simulink library "INT_WESDem_SetPoint"  (R2016b)
settings: Solver=VariableStepAuto  StartTime=0.0  StopTime=10.0  RelTol=1e-3
settings Model: Creator=zhoukai  LastModifiedBy=zhoukai

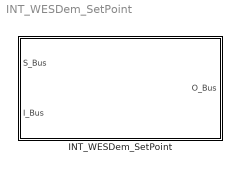
== system INT_WESDem_SetPoint ==
  INT_WESDem_SetPoint : Subsystem

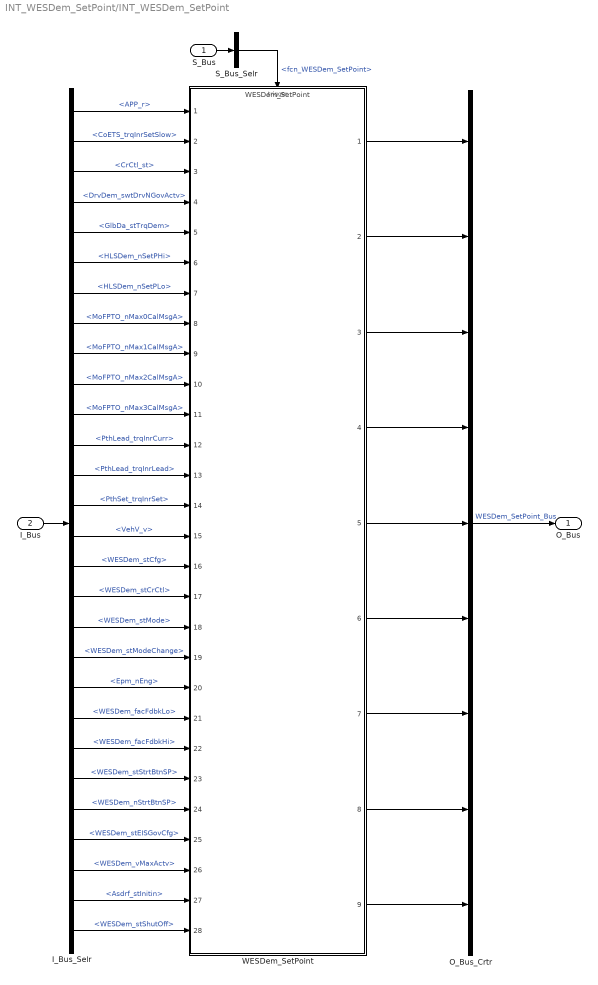
== system INT_WESDem_SetPoint/INT_WESDem_SetPoint ==
  S_Bus : Inport
  I_Bus : Inport  Port=2
  I_Bus_Selr : BusSelector  OutputSignals=APP_r,CoETS_trqInrSetSlow,CrCtl_st,DrvDem_swtDrvNGovActv,GlbDa_stTrqDem,HLSDem_nSetPHi,HLSDem_nSetPLo,MoFPTO_nMax0CalMsgA,MoFPTO_nMax1CalMsgA,MoFPTO_nMax2CalMsgA,MoFPTO_nMax3CalMsgA,PthLead_trqInrCurr,PthLead_trqInrLead,PthSet_trqInrSet,VehV_v,WESDem_stCfg,WESDem_stCrCtl,WESDem_stMode,WESDem_stModeChange,Epm_nEng,WESDem_facFdbkLo,WESDem_facFdbkHi,WESDem_stStrtBtnSP,WESDem_nStrtBtnSP,WESDem_stEISGovCfg,WESDem_vMaxActv,Asdrf_stInitin,WESDem_stShutOff
  O_Bus_Crtr : BusCreator  Inputs=9
  S_Bus_Selr : BusSelector  OutputSignals=fcn_WESDem_SetPoint
  WESDem_SetPoint : ModelReference  ModelNameDialog=WESDem_SetPoint  SimulationMode=Normal  ModelReferenceVersion=1.109  TriggerPortName=function  TriggerPortTriggerType=function-call  TriggerPortStatesWhenEnabling=held
  O_Bus : Outport
  wires:
  S_Bus_Selr/1 -> WESDem_SetPoint/Trigger  "<fcn_WESDem_SetPoint>"
  S_Bus/1 -> S_Bus_Selr/1
  I_Bus/1 -> I_Bus_Selr/1
  I_Bus_Selr/1 -> WESDem_SetPoint/1  "<APP_r>"
  I_Bus_Selr/2 -> WESDem_SetPoint/2  "<CoETS_trqInrSetSlow>"
  I_Bus_Selr/3 -> WESDem_SetPoint/3  "<CrCtl_st>"
  I_Bus_Selr/4 -> WESDem_SetPoint/4  "<DrvDem_swtDrvNGovActv>"
  I_Bus_Selr/5 -> WESDem_SetPoint/5  "<GlbDa_stTrqDem>"
  I_Bus_Selr/6 -> WESDem_SetPoint/6  "<HLSDem_nSetPHi>"
  I_Bus_Selr/7 -> WESDem_SetPoint/7  "<HLSDem_nSetPLo>"
  I_Bus_Selr/8 -> WESDem_SetPoint/8  "<MoFPTO_nMax0CalMsgA>"
  I_Bus_Selr/9 -> WESDem_SetPoint/9  "<MoFPTO_nMax1CalMsgA>"
  I_Bus_Selr/10 -> WESDem_SetPoint/10  "<MoFPTO_nMax2CalMsgA>"
  I_Bus_Selr/11 -> WESDem_SetPoint/11  "<MoFPTO_nMax3CalMsgA>"
  I_Bus_Selr/12 -> WESDem_SetPoint/12  "<PthLead_trqInrCurr>"
  I_Bus_Selr/13 -> WESDem_SetPoint/13  "<PthLead_trqInrLead>"
  I_Bus_Selr/14 -> WESDem_SetPoint/14  "<PthSet_trqInrSet>"
  I_Bus_Selr/15 -> WESDem_SetPoint/15  "<VehV_v>"
  I_Bus_Selr/16 -> WESDem_SetPoint/16  "<WESDem_stCfg>"
  I_Bus_Selr/17 -> WESDem_SetPoint/17  "<WESDem_stCrCtl>"
  I_Bus_Selr/18 -> WESDem_SetPoint/18  "<WESDem_stMode>"
  I_Bus_Selr/19 -> WESDem_SetPoint/19  "<WESDem_stModeChange>"
  I_Bus_Selr/20 -> WESDem_SetPoint/20  "<Epm_nEng>"
  I_Bus_Selr/21 -> WESDem_SetPoint/21  "<WESDem_facFdbkLo>"
  I_Bus_Selr/22 -> WESDem_SetPoint/22  "<WESDem_facFdbkHi>"
  I_Bus_Selr/23 -> WESDem_SetPoint/23  "<WESDem_stStrtBtnSP>"
  I_Bus_Selr/24 -> WESDem_SetPoint/24  "<WESDem_nStrtBtnSP>"
  I_Bus_Selr/25 -> WESDem_SetPoint/25  "<WESDem_stEISGovCfg>"
  I_Bus_Selr/26 -> WESDem_SetPoint/26  "<WESDem_vMaxActv>"
  I_Bus_Selr/27 -> WESDem_SetPoint/27  "<Asdrf_stInitin>"
  I_Bus_Selr/28 -> WESDem_SetPoint/28  "<WESDem_stShutOff>"
  O_Bus_Crtr/1 -> O_Bus/1  "WESDem_SetPoint_Bus"
  WESDem_SetPoint/1 -> O_Bus_Crtr/1
  WESDem_SetPoint/2 -> O_Bus_Crtr/2
  WESDem_SetPoint/3 -> O_Bus_Crtr/3
  WESDem_SetPoint/4 -> O_Bus_Crtr/4
  WESDem_SetPoint/5 -> O_Bus_Crtr/5
  WESDem_SetPoint/6 -> O_Bus_Crtr/6
  WESDem_SetPoint/7 -> O_Bus_Crtr/7
  WESDem_SetPoint/8 -> O_Bus_Crtr/8
  WESDem_SetPoint/9 -> O_Bus_Crtr/9
